simulink library "custom_lib"  (R2015b)
settings: Solver=VariableStepAuto  StartTime=0.0  StopTime=10.0  RelTol=1e-3
settings Model: Creator=valentin_riviere  LastModifiedBy=valentin_riviere

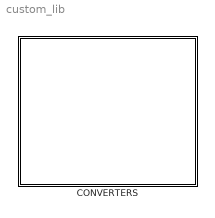
== system custom_lib ==
  CONVERTERS : Subsystem

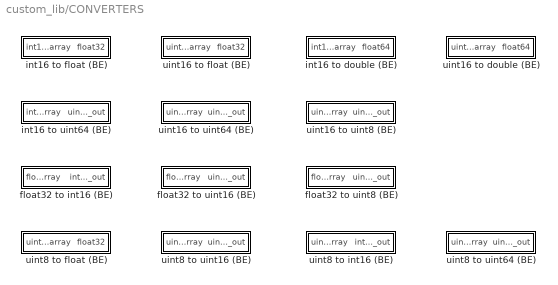
== system custom_lib/CONVERTERS ==
  float32 to int16 (BE) : MATLAB Function  RequirementInfo={} %GIDa_641c6e07_2192_4008_a173_30cc13a99b8d  TreatAsAtomicUnit=on
  float32 to uint16 (BE) : MATLAB Function  RequirementInfo={} %GIDa_6ade4556_beb6_43cd_a7ed_6399e5dc1df2  TreatAsAtomicUnit=on
  float32 to uint8 (BE) : MATLAB Function  RequirementInfo={} %GIDa_6284cd04_ff8b_44bb_96da_c12991b634c6  TreatAsAtomicUnit=on
  int16 to double (BE) : MATLAB Function  RequirementInfo={} %GIDa_eeb816b6_8d0a_4dd1_a2e0_31e478f200c9  TreatAsAtomicUnit=on
  int16 to float (BE) : MATLAB Function  RequirementInfo={} %GIDa_a2f87361_6ebf_4229_8199_5367e1096c87  TreatAsAtomicUnit=on
  int16 to uint64 (BE) : MATLAB Function  RequirementInfo={} %GIDa_9f9f624f_7660_4497_b41b_902332c4cd7e  TreatAsAtomicUnit=on
  uint16 to double (BE) : MATLAB Function  TreatAsAtomicUnit=on
  uint16 to float (BE) : MATLAB Function  TreatAsAtomicUnit=on
  uint16 to uint64 (BE) : MATLAB Function  RequirementInfo={} %GIDa_ef95faaa_e5d6_4a60_bbc2_de1b4a7a313a  TreatAsAtomicUnit=on
  uint16 to uint8 (BE) : MATLAB Function  RequirementInfo={} %GIDa_32be9e63_92b6_4442_9983_553cf8b49b16  TreatAsAtomicUnit=on
  uint8 to float (BE) : MATLAB Function  RequirementInfo={} %GIDa_f69fde1f_901e_42eb_9860_7db15001ba4f  TreatAsAtomicUnit=on
  uint8 to int16 (BE) : MATLAB Function  RequirementInfo={} %GIDa_d203bfc0_ba5c_415c_bbbc_2c1c6c2e1d60  TreatAsAtomicUnit=on
  uint8 to uint16 (BE) : MATLAB Function  RequirementInfo={} %GIDa_f0b88998_baab_4e07_aa61_5740fbc9603e  TreatAsAtomicUnit=on
  uint8 to uint64 (BE) : MATLAB Function  RequirementInfo={} %GIDa_919e84bd_1488_4fa5_bbb1_dd805499e450  TreatAsAtomicUnit=on

== matlab function custom_lib/CONVERTERS/int16 to float (BE) ==
  data: int16_array input int16; float32 output single
function float32 = int16_2_float32_BE(int16_array)
% Convert int16 array (first byte is MSB / Big Endian) to float32

if mod(length(int16_array),2) ~= 0
    error('int16_2_float32_BE : Input length must be even');
else
    float32 = single(zeros(length(int16_array)/2,1));

    for i=1:length(int16_array)/2
        bytepack = int32(int16_array(i));
        bytepack = bitshift(bytepack,16);
        bytepack = bitor(bytepack,bitand(65535,int32(int16_array(i+1))));
        float32(i) = typecast(bytepack,'single');
    end
end

== matlab function custom_lib/CONVERTERS/int16 to uint64 (BE) ==
  data: int16_array input int16; uint64_out output uint64
function uint64_out = int16_2_uint64_BE(int16_array)
% Convert int16 array (first byte is MSB / Big Endian) to uint64

if mod(length(int16_array),4) ~= 0
    error('int16_2_uint64_BE : Input length must multiple of 4');
else
    uint64_out = uint64(zeros(length(int16_array)/4,1));

    for i=1:length(int16_array)/4
        bytepack = bitshift(int64(int16_array(i)),16);
        bytepack = bitshift(bitor(bytepack,bitand(int64(int16_array(i+1)),65535)),16);
        bytepack = bitshift(bitor(bytepack,bitand(int64(int16_array(i+2)),65535)),16);
        uint64_out(i) = bitor(bytepack,bitand(int64(int16_array(i+3)),65535));
    end
end

== matlab function custom_lib/CONVERTERS/uint16 to float (BE) ==
  data: uint16_array input uint16; float32 output single
function float32 = int16_2_float32_BE(uint16_array)
% Convert int16 array (first byte is MSB / Big Endian) to float32

if mod(length(uint16_array),2) ~= 0
    error('int16_2_float32_BE : Input length must be even');
else
    float32 = single(zeros(length(uint16_array)/2,1));

    for i=1:length(uint16_array)/2
        bytepack = int32(uint16_array(i));
        bytepack = bitshift(bytepack,16);
        bytepack = bitor(bytepack,int32(uint16_array(i+1)));
        float32(i) = typecast(bytepack,'single'); 
    end
end

== matlab function custom_lib/CONVERTERS/uint16 to uint64 (BE) ==
  data: uint16_array input uint16; uint64_out output
function uint64_out = uint16_2_uint64_BE(uint16_array)
% Convert uint16 array (first byte is MSB / Big Endian) to uint64

if mod(length(uint16_array),4) ~= 0
    error('uint16_2_uint64_BE : Input length must multiple of 4');
else
    uint64_out = uint64(zeros(length(uint16_array)/4,1));

    for i=1:length(uint16_array)/4
        bytepack = bitshift(int64(uint16_array(i)),16);
        bytepack = bitshift(bitor(bytepack,int64(uint16_array(i+1))),16);
        bytepack = bitshift(bitor(bytepack,int64(uint16_array(i+2))),16);
        uint64_out(i) = bitor(bytepack,int64(uint16_array(i+3)));
    end
end

== matlab function custom_lib/CONVERTERS/int16 to double (BE) ==
  data: int16_array input int16; float64 output double
function float64 = int16_2_float64_BE(int16_array)
% Convert int16 array (first byte is MSB / Big Endian) to float64

if mod(length(int16_array),4) ~= 0
    error('int16_2_float64_BE : Input length must be multiple of 4');
else
    float64 = double(zeros(length(int16_array)/4,1));

    for i=1:length(int16_array)/4
        bytepack = bitshift(int64(int16_array(i)),16);
        bytepack = bitshift(bitor(bytepack,bitand(int64(int16_array(i+1)),65535)),16);
        bytepack = bitshift(bitor(bytepack,bitand(int64(int16_array(i+2)),65535)),16);
        bytepack = bitor(bytepack,bitand(int64(int16_array(i+3)),65535));
        float64(i) = typecast(bytepack,'double'); 
    end
end

== matlab function custom_lib/CONVERTERS/uint16 to double (BE) ==
  data: uint16_array input uint16; float64 output double
function float64 = uint16_2_float64_BE(uint16_array)
% Convert uint16 array (first byte is MSB / Big Endian) to float64

if mod(length(uint16_array),4) ~= 0
    error('uint16_2_float64_BE : Input length must be multiple of 4');
else
    float64 = double(zeros(length(uint16_array)/4,1));

    for i=1:length(uint16_array)/4
        bytepack = bitshift(int64(uint16_array(i)),16);
        bytepack = bitshift(bitor(bytepack,int64(uint16_array(i+1))),16);
        bytepack = bitshift(bitor(bytepack,int64(uint16_array(i+2))),16);
        bytepack = bitor(bytepack,int64(uint16_array(i+3)));
        float64(i) = typecast(bytepack,'double'); 
    end
end

== matlab function custom_lib/CONVERTERS/float32 to int16 (BE) ==
  data: float32_array input single; int16_out output int16
function int16_out = float32_2_int16_BE(float32_array)
% Convert float32 array (first byte is MSB / Big Endian) to int16

    int16_out = single(zeros(length(float32_array)*2,1));

    for i=1:length(float32_array)
        int16_out(2*i:-1:2*i-1) = typecast(single(float32_array(i)),'int16');
    end
end

== matlab function custom_lib/CONVERTERS/float32 to uint16 (BE) ==
  data: float32_array input single; uint16_out output uint16
function uint16_out = float32_2_uint16_BE(float32_array)
% Convert float32 array (first byte is MSB / Big Endian) to uint16

    uint16_out = single(zeros(length(float32_array)*2,1));

    for i=1:length(float32_array)
        uint16_out(2*i:-1:2*i-1) = typecast(single(float32_array(i)),'uint16');
    end
end

== matlab function custom_lib/CONVERTERS/uint8 to float (BE) ==
  data: uint8_array input uint8; float32 output single
function float32 = uint8_2_float32_BE(uint8_array)
% Convert uint8 array (first byte is MSB / Big Endian) to float32

if mod(length(uint8_array),4) ~= 0
    error('uint8_2_float32_BE : Input length must be multpile of 4');
else
    float32 = single(zeros(length(uint8_array)/4,1));

    for i=1:length(float32)
        float32(i) = typecast( bitshift(uint32(uint8_array(4*(i-1)+1)),24)+bitshift(uint32(uint8_array(4*(i-1)+2)),16)+bitshift(uint32(uint8_array(4*(i-1)+3)),8)+uint32(uint8_array(4*(i-1)+4)),'single');
    end
end

== matlab function custom_lib/CONVERTERS/uint8 to uint16 (BE) ==
  data: uint8_array input uint8; uint16_out output single
function uint16_out = uint8_2_uint16_BE(uint8_array)
% Convert uint8 array (first byte is MSB / Big Endian) to uint16

if mod(length(uint8_array),2) ~= 0
    error('uint8_2_uint16_BE : Input length must be multpile of 2');
else
    uint16_out = single(zeros(length(uint8_array)/2,1));

    for i=1:length(uint16_out)
        uint16_out(i) = bitshift(uint16(uint8_array(2*(i-1)+1)),8)+uint16(uint8_array(2*(i-1)+2));
    end
end

== matlab function custom_lib/CONVERTERS/uint8 to int16 (BE) ==
  data: uint8_array input uint8; int16_out output single
function int16_out = uint8_2_int16_BE(uint8_array)
% Convert uint8 array (first byte is MSB / Big Endian) to int16

if mod(length(uint8_array),2) ~= 0
    error('uint8_2_uint16_BE : Input length must be multpile of 2');
else
    int16_out = single(zeros(length(uint8_array)/2,1));

    for i=1:length(int16_out)
        int16_out(i) = typecast(bitshift(uint16(uint8_array(2*(i-1)+1)),8)+uint16(uint8_array(2*(i-1)+2)),'int16');
    end
end

== matlab function custom_lib/CONVERTERS/uint8 to uint64 (BE) ==
  data: uint8_array input uint8; uint64_out output
function uint64_out = uint8_2_uint64_BE(uint8_array)
% Convert uint8 array (first byte is MSB / Big Endian) to uint64

if mod(length(uint8_array),8) ~= 0
    error('uint8_2_uint64_BE : Input length must be multpile of 8');
else
    uint64_out = uint64(zeros(length(uint8_array)/8,1));

    for i=1:length(uint64_out)
        uint64_out(i) = bitshift(uint64(uint8_array(8*(i-1)+1)),56)+bitshift(uint64(uint8_array(8*(i-1)+2)),48)+bitshift(uint64(uint8_array(8*(i-1)+3)),40)+bitshift(uint64(uint8_array(8*(i-1)+4)),32)+bitshift(uint64(uint8_array(8*(i-1)+5)),24)+bitshift(uint64(uint8_array(8*(i-1)+6)),16)+bitshift(uint64(uint8_array(8*(i-1)+7)),8)+uint64(uint8_array(8*(i-1)+8));
    end
end

== matlab function custom_lib/CONVERTERS/float32 to uint8 (BE) ==
  data: float32_array input single; uint8_out output uint8
function uint8_out = float32_2_uint8_BE(float32_array)
% Convert float32 array (first byte is MSB / Big Endian) to uint8

    uint8_out = uint8(zeros(length(float32_array)*4,1));

    for i=1:length(float32_array)
        uint8_out(4*i:-1:4*i-3) = typecast(single(float32_array(i)),'uint8');
    end
end

== matlab function custom_lib/CONVERTERS/uint16 to uint8 (BE) ==
  data: uint16_array input uint16; uint8_out output uint8
function uint8_out = uint16_2_uint8_BE(uint16_array)
% Convert uint16 array (first byte is MSB / Big Endian) to uint8

    uint8_out = uint8(zeros(length(uint16_array)*2,1));

    for i=1:length(uint16_array)
        uint8_out(2*i:-1:2*i-1) = typecast(uint16_array(i),'uint8');
    end
end
